simulink model "milipede_model"  (R2020b)
settings: Solver=FixedStepAuto  StartTime=0.0  StopTime=10.0  FixedStep=.001  MaxStep=.001  RelTol=1e-3  AbsTol=1e-3  EnableMultiTasking=on
values from neighbouring files (symbols this model uses):
  ground_length = 50    [milipede_params.m]
  ground_width = 10    [milipede_params.m]
undefined symbols (not defined in the file or in its folder): sigbuilder_block, X, Y, Z
libraries: nesl_utility x7, sm_lib x4
settings Model: Creator=theaw  LastModifiedBy=theaw
settings SolverCC: AutoScaleAbsTol=off
settings DataIOCC: LimitDataPoints=on  MaxDataPoints=10000
settings OptimizationCC: LifeSpan=inf
settings DebuggingCC: AllowSymbolicDim=off  SFUnexpectedBacktrackingDiag=warning  SFNoUnconditionalDefaultTransitionDiag=warning  SFExecutionAtInitializationDiag=none  ArithmeticOperatorsInVariantConditions=warning
settings SFSimCC: SimUseLocalCustomCode=off  CustomCodeUndefinedFunction=UseInterfaceOnly
settings RTWCC: RTWUseLocalCustomCode=off
settings CodeAppCC: StateflowObjectComments=on
settings GRTTargetCC: TargetLangStandard=C89/C90 (ANSI)
settings ConfigComp: CovMetricSettings=dw  CovSaveCumulativeToWorkspaceVar=on  CovSaveSingleToWorkspaceVar=on  CovExternalEMLEnable=off  CovSFcnEnable=off
settings SimscapeCC: SimscapeLogType=all  SimscapeLogSimulationStatistics=on  SimscapeLogDataHistory=10000

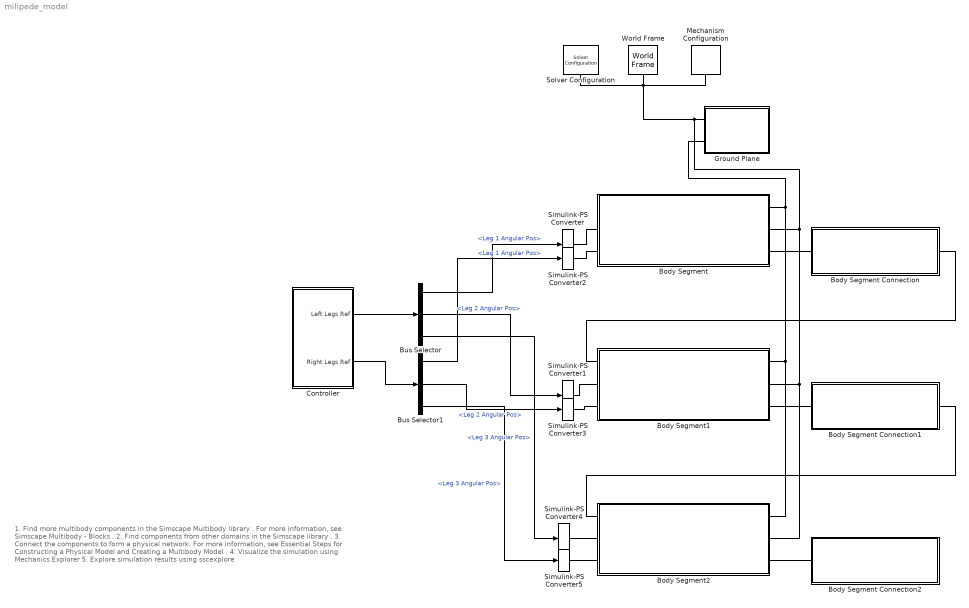
== system milipede_model ==
  note: 1. Find more multibody components in the Simscape Multibody library .
      | For more information, see Simscape Multibody - Blocks .
      | 2. Find components from other domains in the Simscape library .
      | 3. Connect the components to form a physical network.
      | For more information, see Essential Steps for Constructing a Physical Model and Creating a Multibody Model .
      | 4. Visualize the simulation using Mechanics Explorer
      | 5. Explore simulation results using sscexplore
  Body Segment : Subsystem  ReferencedSubsystem=Body_Segment
      settings: PortSchema="{\"entries\":[{\"content\":{\"sides\":[{\"content\":{\"connectorIds\":[\"LConn2\",\"LConn4\",\"LConn5\"]},\"type\":\"ConnectorPlacement.EquallySpacedRectSide\",\"uuid\":\"fb737d30-ca9f-4a68-95a5-e3a7ce86cb45\"},{\"content\":{\"connectorIds\":[\"LConn1\",\"LConn3\",\"RConn1\"],\"side\":\"RIGHT\"},\"type\":\"ConnectorPlacement.EquallySpacedRectSide\",\"uuid\":\"539e621e-5113-4794-9972-87c15e98d4d9\"},{\"content\":{\"connectorIds\":[],\"side\":\"TOP\"},\"type\":\"ConnectorPlacement.EquallySpacedRectSide\",\"uuid\":\"8962975b-bd6e-4d1d-985a-26c257813034\"},{\"content\":{\"connectorIds\":[],\"side\":\"HIDDEN\"},\"type\":\"ConnectorPlacement.EquallySpacedRectSide\",\"uuid\":\"77212b56-7770-4821-8d47-cbc5f5c7ad4e\"}]},\"type\":\"ConnectorPlacement.EquallySpacedConnector\",\"uuid\":\"df3cce63-7ff8-4f52-99d5-50b9183cdf40\"}],\"packageUris\":[\"http://schema.mathworks.com/mf0/Connector/R2020b\"],\"version\":\"1.0\"}"
  Body Segment Connection : Subsystem  ReferencedSubsystem=Body_Segment_Connection
  Body Segment Connection1 : Subsystem  ReferencedSubsystem=Body_Segment_Connection
  Body Segment Connection2 : Subsystem  ReferencedSubsystem=Body_Segment_Connection
  Body Segment1 : Subsystem  ReferencedSubsystem=Body_Segment
      settings: PortSchema="{\"entries\":[{\"content\":{\"sides\":[{\"content\":{\"connectorIds\":[\"LConn2\",\"LConn4\",\"LConn5\"]},\"type\":\"ConnectorPlacement.EquallySpacedRectSide\",\"uuid\":\"fb737d30-ca9f-4a68-95a5-e3a7ce86cb45\"},{\"content\":{\"connectorIds\":[\"LConn1\",\"LConn3\",\"RConn1\"],\"side\":\"RIGHT\"},\"type\":\"ConnectorPlacement.EquallySpacedRectSide\",\"uuid\":\"539e621e-5113-4794-9972-87c15e98d4d9\"},{\"content\":{\"connectorIds\":[],\"side\":\"TOP\"},\"type\":\"ConnectorPlacement.EquallySpacedRectSide\",\"uuid\":\"8962975b-bd6e-4d1d-985a-26c257813034\"},{\"content\":{\"connectorIds\":[],\"side\":\"HIDDEN\"},\"type\":\"ConnectorPlacement.EquallySpacedRectSide\",\"uuid\":\"77212b56-7770-4821-8d47-cbc5f5c7ad4e\"}]},\"type\":\"ConnectorPlacement.EquallySpacedConnector\",\"uuid\":\"df3cce63-7ff8-4f52-99d5-50b9183cdf40\"}],\"packageUris\":[\"http://schema.mathworks.com/mf0/Connector/R2020b\"],\"version\":\"1.0\"}"
  Body Segment2 : Subsystem  ReferencedSubsystem=Body_Segment
      settings: PortSchema="{\"entries\":[{\"content\":{\"sides\":[{\"content\":{\"connectorIds\":[\"LConn2\",\"LConn4\",\"LConn5\"]},\"type\":\"ConnectorPlacement.EquallySpacedRectSide\",\"uuid\":\"fb737d30-ca9f-4a68-95a5-e3a7ce86cb45\"},{\"content\":{\"connectorIds\":[\"LConn1\",\"LConn3\",\"RConn1\"],\"side\":\"RIGHT\"},\"type\":\"ConnectorPlacement.EquallySpacedRectSide\",\"uuid\":\"539e621e-5113-4794-9972-87c15e98d4d9\"},{\"content\":{\"connectorIds\":[],\"side\":\"TOP\"},\"type\":\"ConnectorPlacement.EquallySpacedRectSide\",\"uuid\":\"8962975b-bd6e-4d1d-985a-26c257813034\"},{\"content\":{\"connectorIds\":[],\"side\":\"HIDDEN\"},\"type\":\"ConnectorPlacement.EquallySpacedRectSide\",\"uuid\":\"77212b56-7770-4821-8d47-cbc5f5c7ad4e\"}]},\"type\":\"ConnectorPlacement.EquallySpacedConnector\",\"uuid\":\"df3cce63-7ff8-4f52-99d5-50b9183cdf40\"}],\"packageUris\":[\"http://schema.mathworks.com/mf0/Connector/R2020b\"],\"version\":\"1.0\"}"
  Bus Selector : BusSelector  OutputSignals=Leg 1 Angular Pos,Leg 2 Angular Pos,Leg 3 Angular Pos
  Bus Selector1 : BusSelector  OutputSignals=Leg 1 Angular Pos,Leg 2 Angular Pos,Leg 3 Angular Pos
  Controller : Subsystem
  Ground Plane : Subsystem
  Mechanism Configuration : sm_lib/Utilities/Mechanism Configuration  UniformGravity=Constant  GravityVector=[0 0 -9.80665]  GravityVectorUnits=m/s^2  GravityUnits=m/s^2  LinearizationDelta=0.001  JointModeTransitionNonlinearIterations=2
      settings: SourceProductName=Multibody
  Simulink-PS Converter{,1..5} (6 alike) : nesl_utility/Simulink-PS Converter  PhysicalDomain=network_engine_domain  SubClassName=ps_input  LeftPortType=input  RightPortType=output  PseudoPeriodic=off  Frequencies=[]  NoiseDistribution=none  NoiseParameters=[]  Unit=rad  AffineConversion=off  FilteringAndDerivatives=filter  SimscapeFilterOrder=2  InputFilterTimeConstant=0.001  UdotUserProvided=2
  Solver Configuration : nesl_utility/Solver Configuration  PhysicalDomain=network_engine_domain  SubClassName=solver  LeftPortType=input  RightPortType=generic  Tones=[]  Harmonics=[]  SimulateNoise=off  Profile=off  UseLocalSampling=off  EnableSwitchedLinearOptims=on  FrequencyDomain=off  UseCCode=off  RelTol=0.001  AbsTol=1e-06  MinStep=1e-09  ToWorkspace=off  RevertToSquareIcSolve=off  NumHomotopyIterations=100  PhasorMode=off  PhasorModeNumHarmonics=1  DoDC=off  ResidualTolerance=1e-09  UseLocalSolver=off  LocalSolverChoice=NE_BACKWARD_EULER_ADVANCER  LocalSolverSampleTime=0.001  DoFixedCost=off  MaxNonlinIter=3  MaxModeIter=2  ComputeImpulses=off  ImpulseIterations=2  LinearAlgebra=Sparse  EquationFormulation=NE_TIME_EF  DelaysMemoryBudget=1024  AutomaticFiltering=on  FilteringTimeConstant=0.001  PartitionStorageMethod=AS_NEEDED  PartitionMemoryBudget=1024  PartitionMethod=FAST
      settings: SourceProductName=Utilities
  World Frame : sm_lib/Frames and Transforms/World Frame
      settings: SourceProductName=Multibody
  wires:
  Controller/1(Left Legs Ref) -> Bus Selector/1
  Controller/2(Right Legs Ref) -> Bus Selector1/1
  Bus Selector/1 -> Simulink-PS Converter/1  "<Leg 1 Angular Pos>"
  Bus Selector1/1 -> Simulink-PS Converter2/1  "<Leg 1 Angular Pos>"
  Bus Selector/2 -> Simulink-PS Converter1/1  "<Leg 2 Angular Pos>"
  Bus Selector/3 -> Simulink-PS Converter4/1  "<Leg 3 Angular Pos>"
  Bus Selector1/2 -> Simulink-PS Converter3/1  "<Leg 2 Angular Pos>"
  Bus Selector1/3 -> Simulink-PS Converter5/1  "<Leg 3 Angular Pos>"
  connections:
  Simulink-PS Converter/RConn1 -- Body Segment/LConn4
  Solver Configuration/RConn1 -- Body Segment2/LConn3 -- Body Segment1/LConn3 -- Body Segment/LConn3 -- Ground Plane/LConn1 -- Mechanism Configuration/RConn1 -- World Frame/RConn1
  Simulink-PS Converter2/RConn1 -- Body Segment/LConn5
  Body Segment Connection/LConn1 -- Body Segment/RConn1
  Body Segment Connection1/LConn1 -- Body Segment1/RConn1
  Body Segment Connection2/LConn1 -- Body Segment2/RConn1
  Body Segment Connection1/RConn1 -- Body Segment2/LConn2
  Body Segment Connection/RConn1 -- Body Segment1/LConn2
  Body Segment1/LConn1 -- Ground Plane/LConn2 -- Body Segment/LConn1 -- Body Segment2/LConn1
  Body Segment1/LConn5 -- Simulink-PS Converter3/RConn1
  Body Segment1/LConn4 -- Simulink-PS Converter1/RConn1
  Simulink-PS Converter4/RConn1 -- Body Segment2/LConn4
  Simulink-PS Converter5/RConn1 -- Body Segment2/LConn5

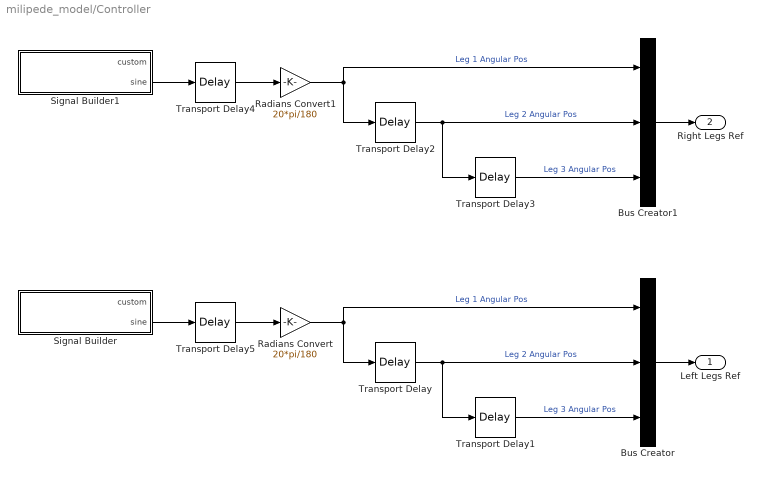
== system milipede_model/Controller ==
  Bus Creator : BusCreator  Inputs=3
  Bus Creator1 : BusCreator  Inputs=3
  Radians Convert : Gain  Gain=20*pi/180
  Radians Convert1 : Gain  Gain=20*pi/180
  Signal Builder : Subsystem  Tag=STV Subsys  LoadFcn=sigbuilder_block('load');  StartFcn=sigbuilder_block('start');  StopFcn=sigbuilder_block('stop');  ClipboardFcn=sigbuilder_block('clipboard');  mask(Sigbuilder block){tuvar=[0:10]}
      mask help: Simulink:masks:SigbuilderBlock_MD
      mask init:
      | if ~strcmp(get_param(bdroot(gcbh),'SimulationStatus'),'stopped') tuvar = sigbuilder_block('maskInit'); end
      settings: CopyFcn=sigbuilder_block('copy');  DeleteFcn=sigbuilder_block('delete');  ModelCloseFcn=sigbuilder_block('modelClose');  PreSaveFcn=sigbuilder_block('preSave');  PauseFcn=sigbuilder_block('pause');  ContinueFcn=sigbuilder_block('continue');  NameChangeFcn=sigbuilder_block('namechange');  OpenFcn=sigbuilder_block('open',[437.6 199.2 550.4 400 ]);  CloseFcn=sigbuilder_block('close');
      mask Display: plot(0, 0, 100, 100,[2, 2, 32, 32, 2], [68, 8, 8, 68, 68],[32, 2], [38, 38], [32, 19, 2],[53, 60, 44], [32, 17, 17, 2],[16, 16, 31, 31]);txt = getActiveGroup(gcbh);text(2, 100, txt,'verticalAlignment', 'top');
  Signal Builder1 : Subsystem  Tag=STV Subsys  LoadFcn=sigbuilder_block('load');  StartFcn=sigbuilder_block('start');  StopFcn=sigbuilder_block('stop');  ClipboardFcn=sigbuilder_block('clipboard');  mask(Sigbuilder block){tuvar=[0:10]}
      mask help: Simulink:masks:SigbuilderBlock_MD
      mask init:
      | if ~strcmp(get_param(bdroot(gcbh),'SimulationStatus'),'stopped') tuvar = sigbuilder_block('maskInit'); end
      settings: CopyFcn=sigbuilder_block('copy');  DeleteFcn=sigbuilder_block('delete');  ModelCloseFcn=sigbuilder_block('modelClose');  PreSaveFcn=sigbuilder_block('preSave');  PauseFcn=sigbuilder_block('pause');  ContinueFcn=sigbuilder_block('continue');  NameChangeFcn=sigbuilder_block('namechange');  OpenFcn=sigbuilder_block('open',[437.6 199.2 550.4 400 ]);  CloseFcn=sigbuilder_block('close');
      mask Display: plot(0, 0, 100, 100,[2, 2, 32, 32, 2], [68, 8, 8, 68, 68],[32, 2], [38, 38], [32, 19, 2],[53, 60, 44], [32, 17, 17, 2],[16, 16, 31, 31]);txt = getActiveGroup(gcbh);text(2, 100, txt,'verticalAlignment', 'top');
  Transport Delay{,1..3,5} (5 alike) : TransportDelay  DelayTime=.338
  Transport Delay4 : TransportDelay  DelayTime=0
  Left Legs Ref : Outport
  Right Legs Ref : Outport  Port=2
  wires:
  Radians Convert/1 -> Bus Creator/1, Transport Delay/1  "Leg 1 Angular Pos"
  Transport Delay/1 -> Transport Delay1/1, Bus Creator/2  "Leg 2 Angular Pos"
  Bus Creator/1 -> Left Legs Ref/1
  Transport Delay1/1 -> Bus Creator/3  "Leg 3 Angular Pos"
  Transport Delay2/1 -> Transport Delay3/1, Bus Creator1/2  "Leg 2 Angular Pos"
  Transport Delay3/1 -> Bus Creator1/3  "Leg 3 Angular Pos"
  Bus Creator1/1 -> Right Legs Ref/1
  Radians Convert1/1 -> Bus Creator1/1, Transport Delay2/1  "Leg 1 Angular Pos"
  Signal Builder1/2(sine) -> Transport Delay4/1
  Transport Delay4/1 -> Radians Convert1/1
  Transport Delay5/1 -> Radians Convert/1
  Signal Builder/2(sine) -> Transport Delay5/1

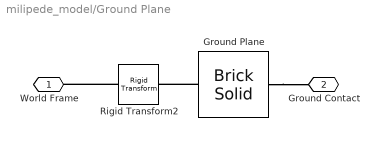
== system milipede_model/Ground Plane ==
  Ground Plane : sm_lib/Body Elements/Brick Solid  GraphicAmbientColor=[0.15 0.15 0.15 1.0]  BasedOnType=Density  BrickDimensions=[ground_width ground_length .5]  BrickDimensionUnits=m  CenterOfMass=[0 0 0]  CenterOfMassUnits=m  GraphicDiffuseColor=[0.0 0.4 0.6]  Density=1000  DensityUnits=kg/m^3  DoExposeReferenceFrame=on  GraphicEmissiveColor=[0.0 0.0 0.0 1.0]  ExportEntireGeometry=on  SerializedFrames=<Frames/>  MarkerShape=Sphere  MarkerSize=10  GraphicType=FromGeometry  InertiaType=CalculateFromGeometry  Mass=1  MassUnits=kg  MomentsOfInertia=[1 1 1]  MomentsOfInertiaUnits=kg*m^2  GraphicOpacity=1.0  ProductsOfInertia=[0 0 0]  ProductsOfInertiaUnits=kg*m^2  GraphicShininess=75  GraphicSpecularColor=[0.5 0.5 0.5 1.0]  GraphicVisPropType=SimpleVisualProperties
  Rigid Transform2 : sm_lib/Frames and Transforms/Rigid Transform  TranslationMethod=StandardAxis  TranslationStandardOffset=ground_plane_z  TranslationLengthUnit=m  TranslationStandardAxis=+Z  TranslationCartesianOffset=[0 0 0]  TranslationROffset=0  TranslationROffsetUnits=m  TranslationZOffset=0  TranslationZOffsetUnits=m  TranslationThetaOffset=0  TranslationThetaOffsetUnits=deg  RotationMethod=None  RotationAngleUnits=deg  RotationStandardAxis=+X  RotationAngle=0  RotationArbitraryAxis=[0 0 1]  FollAlignAxisA=+X  BaseAlignAxisA=+Y  FollAlignAxisB=+Y  BaseAlignAxisB=+Z  RotationSequenceAxes=FollowerAxes  RotationSequence=XYX  RotationSequenceAngles=[0 0 0]  RotationSequenceAnglesUnits=deg  RotationMatrix=[1 0 0; 0 1 0; 0 0 1]
  World Frame : PMIOPort  Side=Left
  Ground Contact : PMIOPort  Port=2  Side=Left
  connections:
  Rigid Transform2/LConn1 -- World Frame/RConn1
  Ground Plane/RConn1 -- Rigid Transform2/RConn1
  Ground Plane/LConn1 -- Ground Contact/RConn1

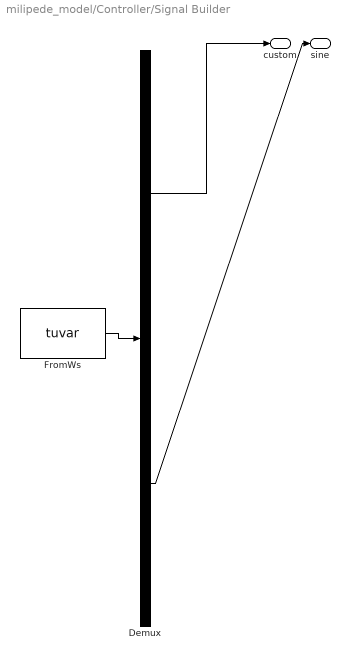
== system milipede_model/Controller/Signal Builder ==
  Demux : Demux  Tag=STV Demux  Outputs=2
      settings: DisplayOption=none
  FromWs : FromWorkspace  Tag=STV FromWs  VariableName=tuvar
      SigBuilderData=|
      | common.afterFinalStr = 'Extrapolate'
      | common.sampleTime = 0
      | dataSet.timeRange = [0 10]
      | dataSet.name = 'Group 1'
      | sbobj.Groups.Name = 'Group 1'
      | sbobj.Groups.Signals(1).Name = 'custom'
      | sbobj.Groups.Signals(1).XData = [0 0.146 0.2 0.25 0.3 0.348 0.5 0.642 0.7 0.75 0.802 0.852 10]
      | sbobj.Groups.Signals(1).YData = [0 0 0.94 1 0.94 0.01 1.22464679915e-16 -0.04 -0.92 -1 -0.93 -0.06 -0.06]
      | sbobj.Groups.Signals(2).Name = 'sine'
      | sbobj.Groups.Signals(2).XData = [0 0.125 0.25 0.375 0.5 0.625 0.75 0.875 1 1.125 1.25 1.375 1.5 1.625 1.75 1.875 2 2.125 2.25 2.375 2.5 2.625 2.75 2.875 3 3.125 3.25 3.375 3.5 3.625 3.75 3.875 4 4.125 4.25 4.375 4.5 4.625 4.75 4.875 5 5.125 5.25 5.375 5.5 5.625 5.75 5.875 6 6.125 6.25 6.375 6.5 6.625 6.75 6.875 7 7.125 7.25 7.375 7.5 7.625 7.75 7.875 8 8.125 8.25 8.375 8.5 8.625 8.75 8.875 9 9.125 9.25 9.375 9.5 9.625 9.75 9.875 10]
      | sbobj.Groups.Signals(2).YData = [0 0.707106781187 1 0.707106781187 1.22464679915e-16 -0.707106781187 -1 -0.707106781187 0 0.707106781187 1 0.707106781187 1.22464679915e-16 -0.707106781187 -1 -0.707106781187 0 0.707106781187 1 0.707106781187 1.22464679915e-16 -0.707106781187 -1 -0.707106781187 0 0.707106781187 1 0.707106781187 1.22464679915e-16 -0.707106781187 -1 -0.707106781187 0 0.707106781187 1 0.707106781187 1.22464679915e-16 -0.707106781187 -1 -0.707106781187 0 0.707106781187 1 0.707106781187 1.22464679915e-16 -0.707106781187 -1 -0.707106781187 0 0.707106781187 1 0.707106781187 1.22464679915e-16 -0.707106781187 -1 -0.707106781187 0 0.707106781187 1 0.707106781187 1.22464679915e-16 -0.707106781187 -1 -0.707106781187 0 0.707106781187 1 0.707106781187 1.22464679915e-16 -0.707106781187 -1 -0.707106781187 0 0.707106781187 1 0.707106781187 1.22464679915e-16 -0.707106781187 -1 -0.707106781187 0]
  custom : Outport  Tag=STV Outport
  sine : Outport  Tag=STV Outport  Port=2
  wires:
  FromWs/1 -> Demux/1
  Demux/1 -> custom/1
  Demux/2 -> sine/1

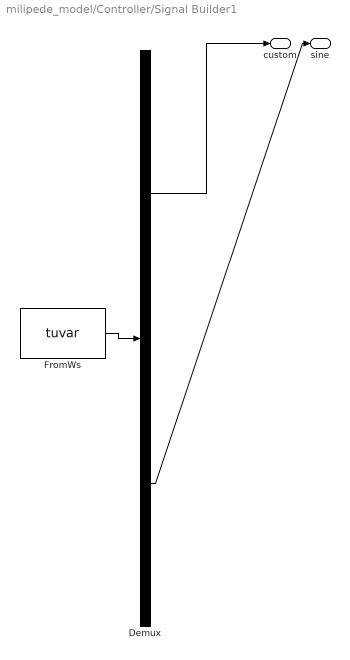
== system milipede_model/Controller/Signal Builder1 ==
  Demux : Demux  Tag=STV Demux  Outputs=2
      settings: DisplayOption=none
  FromWs : FromWorkspace  Tag=STV FromWs  VariableName=tuvar
      SigBuilderData=|
      | common.afterFinalStr = 'Extrapolate'
      | common.sampleTime = 0
      | dataSet.timeRange = [0 10]
      | dataSet.name = 'Group 1'
      | sbobj.Groups.Name = 'Group 1'
      | sbobj.Groups.Signals(1).Name = 'custom'
      | sbobj.Groups.Signals(1).XData = [0 0.146 0.2 0.25 0.3 0.348 0.5 0.642 0.7 0.75 0.802 0.852 10]
      | sbobj.Groups.Signals(1).YData = [0 0 0.94 1 0.94 0.01 1.22464679915e-16 -0.04 -0.92 -1 -0.93 -0.06 -0.06]
      | sbobj.Groups.Signals(2).Name = 'sine'
      | sbobj.Groups.Signals(2).XData = [0 0.125 0.25 0.375 0.5 0.625 0.75 0.875 1 1.125 1.25 1.375 1.5 1.625 1.75 1.875 2 2.125 2.25 2.375 2.5 2.625 2.75 2.875 3 3.125 3.25 3.375 3.5 3.625 3.75 3.875 4 4.125 4.25 4.375 4.5 4.625 4.75 4.875 5 5.125 5.25 5.375 5.5 5.625 5.75 5.875 6 6.125 6.25 6.375 6.5 6.625 6.75 6.875 7 7.125 7.25 7.375 7.5 7.625 7.75 7.875 8 8.125 8.25 8.375 8.5 8.625 8.75 8.875 9 9.125 9.25 9.375 9.5 9.625 9.75 9.875 10]
      | sbobj.Groups.Signals(2).YData = [0 0.707106781187 1 0.707106781187 1.22464679915e-16 -0.707106781187 -1 -0.707106781187 0 0.707106781187 1 0.707106781187 1.22464679915e-16 -0.707106781187 -1 -0.707106781187 0 0.707106781187 1 0.707106781187 1.22464679915e-16 -0.707106781187 -1 -0.707106781187 0 0.707106781187 1 0.707106781187 1.22464679915e-16 -0.707106781187 -1 -0.707106781187 0 0.707106781187 1 0.707106781187 1.22464679915e-16 -0.707106781187 -1 -0.707106781187 0 0.707106781187 1 0.707106781187 1.22464679915e-16 -0.707106781187 -1 -0.707106781187 0 0.707106781187 1 0.707106781187 1.22464679915e-16 -0.707106781187 -1 -0.707106781187 0 0.707106781187 1 0.707106781187 1.22464679915e-16 -0.707106781187 -1 -0.707106781187 0 0.707106781187 1 0.707106781187 1.22464679915e-16 -0.707106781187 -1 -0.707106781187 0 0.707106781187 1 0.707106781187 1.22464679915e-16 -0.707106781187 -1 -0.707106781187 0]
  custom : Outport  Tag=STV Outport
  sine : Outport  Tag=STV Outport  Port=2
  wires:
  FromWs/1 -> Demux/1
  Demux/1 -> custom/1
  Demux/2 -> sine/1
